simulink model "AirVehicle"  (R2026a)
settings: configuration reference "quad_config" (kept outside this file)
undefined symbols (not defined in the file): g, ts_uav
libraries: simulink x1, uavalgslib x1
settings Model: DataDictionary=QuadData.sldd  Creator=The MathWorks, Inc.  LastModifiedBy=The MathWorks, Inc.
settings ConfigSetRef: SourceName=quad_config

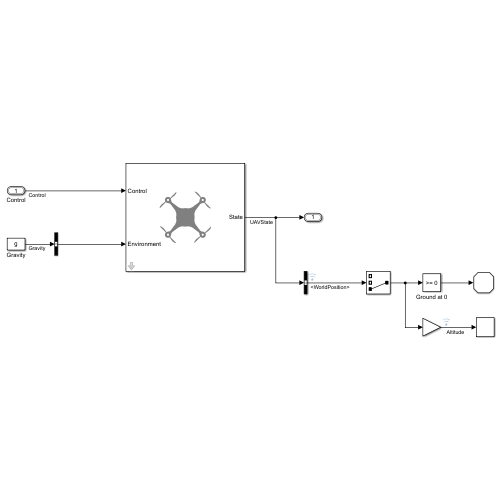
[thumbnail: Simulink's stored preview of the top-level diagram]
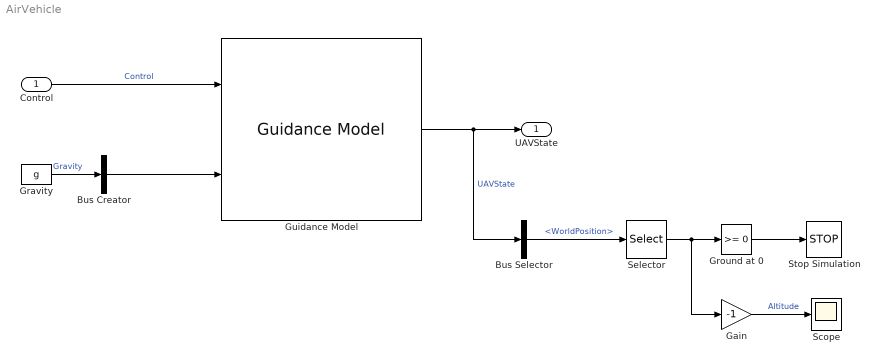
== system AirVehicle ==
  Control : Inport  OutDataTypeStr=Bus: MultirotorGuidanceControlBus  BusOutputAsStruct=on
  Bus Creator : BusCreator  Inputs=1  OutDataTypeStr=Bus: MultirotorGuidanceEnvironmentBus  NonVirtualBus=on
  Bus Selector : BusSelector  OutputSignals=WorldPosition
  Gain : Gain  Gain=-1
  Gravity : Constant  Value=g  SampleTime=ts_uav
  Ground at 0 : simulink/Logic and Bit Operations/Compare To Constant  relop=>=  const=0  OutDataTypeStr=boolean
  Guidance Model : uavalgslib/Guidance Model  ModelType=MultirotorGuidance  NumInstances=1  SpecifiedDataType=double  SimulateUsing=Interpreted execution  InitialWorldPositionMultirotor=[0; 0; -0.1]  InitialWorldVelocityMultirotor=[0; 0; 0]  InitialEulerZYXMultirotor=[0; 0; 0]  InitialBodyAngularRateRPYMultirotor=[0; 0; 0]  InitialThrustMultirotor=0.4905  InitialNorthFixedWing=0  InitialEastFixedWing=0  InitialHeightFixedWing=0  InitialAirSpeedFixedWing=0  InitialHeadingAngleFixedWing=0  InitialFlightPathAngleFixedWing=0  InitialRollAngleFixedWing=0  InitialRollAngleRateFixedWing=0  PDRollMultirotor=[25, 7]  PDPitchMultirotor=[25, 7]  PYawRateMultirotor=25  PThrustMultirotor=25  MassMultirotor=UAVmass  PHeightFixedWing=3.9  PHeadingAngleFixedWing=3.9  PFlightPathAngleFixedWing=39  PDRollFixedWing=[3402.97, 116.67]  PAirSpeedFixedWing=1  FlightPathAngleLimitsFixedWing=[-pi/2, pi/2]  StateBusName='MultirotorGuidanceStateBus'  ControlBusName='MultirotorGuidanceControlBus'  EnvironmentBusName='MultirotorGuidanceEnvironmentBus'  DataType=double
  Scope : Scope
  Selector : Selector  InputPortWidth=3  IndexOptions=Index vector (dialog)  Indices=3  OutputSizes=1
  Stop Simulation : Stop
  UAVState : Outport  OutDataTypeStr=Bus: MultirotorGuidanceStateBus
  wires:
  Guidance Model/1 -> UAVState/1, Bus Selector/1  "UAVState"
  Gravity/1 -> Bus Creator/1  "Gravity"
  Bus Creator/1 -> Guidance Model/2
  Control/1 -> Guidance Model/1  "Control"
  Bus Selector/1 -> Selector/1  "<WorldPosition>"
  Selector/1 -> Ground at 0/1, Gain/1
  Ground at 0/1 -> Stop Simulation/1
  Gain/1 -> Scope/1  "Altitude"
